simulink model "Progetto"  (R2022b)
settings: Solver=FixedStepDiscrete  StartTime=0.0  StopTime=10.0  FixedStep=0.1  RelTol=1e-3
InitFcn:
  | mbd_s32k_consistency_checks(bdroot(gcs));
libraries: simulink x1, mbd_s32k1xx_ec_toolbox x1
settings Model: Creator=marpe  LastModifiedBy=marpe
settings DataIOCC: ExternalInput=off  InitialState=off  SaveOutput=off  SignalLogging=off  SaveTime=off
settings OptimizationCC: DefaultParameterBehavior=Inlined  EnhancedBackFolding=on  PassReuseOutputArgsAs=Individual arguments  ZeroExternalMemoryAtStartup=off  ZeroInternalMemoryAtStartup=off  OptimizeBlockOrder=speed  DifferentSizesBufferReuse=on  OptimizationCustomize=off  EfficientTunableParamExpr=on
settings DebuggingCC: InheritedTsInSrcMsg=none  SingleTaskRateTransMsg=error  ParameterTunabilityLossMsg=error  UnconnectedInputMsg=error  UnconnectedOutputMsg=error  UnconnectedLineMsg=error  UnknownTsInhSupMsg=error
settings HardwareCC: ProdBitPerPointer=32  ProdBitPerSizeT=32  ProdBitPerPtrDiffT=32  ProdLargestAtomicInteger=Long  ProdLargestAtomicFloat=Double  ProdWordSize=32  ProdHWDeviceType=ARM Compatible->ARM Cortex
settings ModelReferenceCC: ModelReferenceNumInstancesAllowed=Single  PropagateVarSize=During execution
settings SFSimCC: MATLABDynamicMemAlloc=off
settings RTWCC: Description=Model Based Design Toolbox S32K1xx Code Generation Target  SystemTargetFile=mbd_s32k.tlc  MakeCommand=mbd_s32k_make_rtw COPY_MDLREF_INCLUDES=0  TemplateMakefile=mbd_s32k.tmf  GenerateReport=on  LaunchReport=on  GenerateWebview=on
settings CodeAppCC: ForceParamTrailComments=on  IgnoreCustomStorageClasses=off  OperatorAnnotations=on  SimulinkDataObjDesc=on  SFDataObjDesc=on  InsertBlockDesc=on
settings STFCustomTargetCC: TargetLangStandard=C99 (ISO)  MultiwordLength=256  CombineOutputUpdateFcns=on  ERTCustomFileBanners=on  SupportContinuousTime=off  SupportNonInlinedSFcns=off  RemoveResetFunc=on  SupportVariableSizeSignals=on  MATLABClassNameForMDSCustomization=Simulink.SoftwareTarget.ERTCustomization  SystemTargetFile=mbd_s32k.tlc
settings ERTTargetCC: TargetLangStandard=C99 (ISO)  ParMdlRefBuildCompliant=off  CompOptLevelCompliant=off  ConcurrentExecutionCompliant=off  SupportVariableSizeSignals=on  ModelStepFunctionPrototypeControlCompliant=off  CPPClassGenCompliant=off  UseToolchainInfoCompliant=off  InlinedParameterPlacement=NonHierarchical  ERTSrcFileBannerTemplate=mbd_ert_code_template.cgt  ERTHdrFileBannerTemplate=mbd_ert_code_template.cgt  ERTDataSrcFileTemplate=mbd_ert_code_template.cgt  ERTDataHdrFileTemplate=mbd_ert_code_template.cgt  ERTCustomFileTemplate=example_file_process.tlc

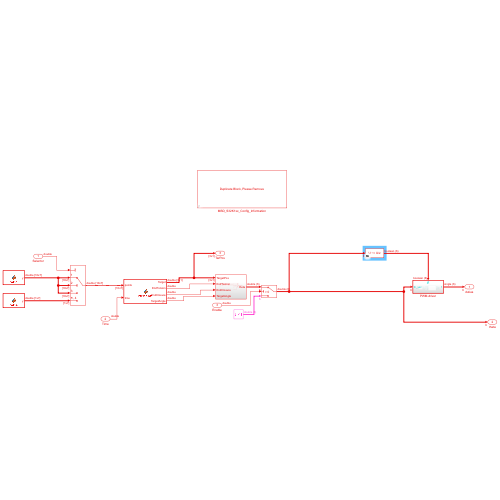
[thumbnail: Simulink's stored preview of the top-level diagram]
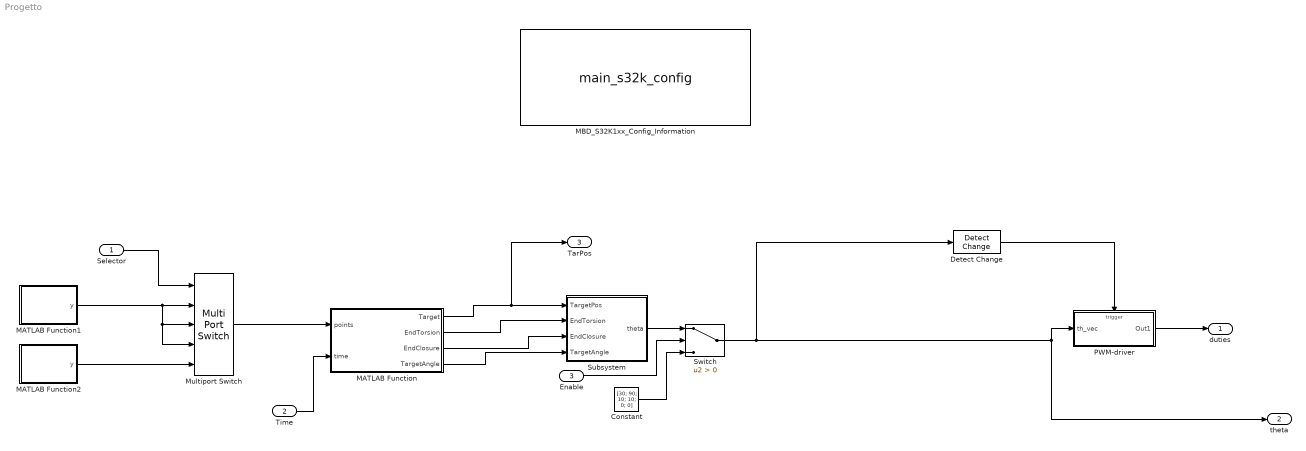
== system Progetto ==
  Selector : Inport  PortDimensions=1
  Time : Inport  Port=2  PortDimensions=1
  Enable : Inport  Port=3
  Constant : Constant  Value=[30; 90; 10; 10; 0; 0]
  Detect Change : simulink/Logic and Bit Operations/Detect Change  vinit=[0; 0; 0; 0; 0; 0]  OutDataTypeStr=boolean
  MATLAB Function : MATLAB Function  TreatAsAtomicUnit=on
  MATLAB Function1 : MATLAB Function  TreatAsAtomicUnit=on
  MATLAB Function2 : MATLAB Function  TreatAsAtomicUnit=on
  MBD_S32K1xx_Config_Information : S-Function  AncestorBlock=mbd_s32k1xx_ec_toolbox/MBD_S32K1xx_Config_Information  LoadFcn=|  InitFcn=|  FunctionName=main_s32k_config  SFunctionDeploymentMode=off  EnableBusSupport=off  mask(MBDTBX_EC_S32K){mbdt_ver=0, disp_str=|, config_params=[], mcu_target_name=S32K144, mcu_target_package=100-LQFP, mcu_target_sram_size=48KB, mcu_system_clock_freq=80, mcu_xtal_freq=External 8, mcu_steptick_timer=LPIT Channel 0, mcu_steptick_prio=15, ds_import_enable=on, target_compiler=GCC, target_memory=FLASH, gcc_target_compile_opts=-mthumb -mfloat-abi=hard -mfpu=fpv4-sp-d16 -O1 -g -gstrict-dwarf, gcc_target_assemble_opts=-mthumb -mfloat-abi=hard -mfpu=fpv4-sp-d16 -g, gcc_target_link_opts=-mthumb -mfloat-abi=hard -mfpu=fpv4-sp-d16, gcc_target_lib_opts=, gcc_target_default_lcf=on, gcc_target_user_lcf=S32K144_48_flash.ld, ghs_target_compile_opts=-cpu=cortexm4f -thumb -fpu=vfpv4_d16 -fsingle -Ogeneral -Wundef -Wimplicit-int -Wshadow -Wtrigraphs --no_commons --gnu_asm -gnu99 -gdwarf-2 -G, ghs_target_assemble_opts=-cpu=cortexm4f -fpu=vfpv4_d16, ghs_target_link_opts=-cpu=cortexm4f -thumb -fpu=vfpv4_d16, ghs_target_lib_opts=, ghs_target_default_lcf=on, ghs_target_user_lcf=S32K144_48_flash.ld, iar_target_compile_opts=--cpu=Cortex-M4F --thumb --fpu=VFPv4_sp -Ol -e --debug --dlib_config normal, iar_target_assemble_opts=--cpu Cortex-M4F --thumb --fpu VFPv4_sp, iar_target_link_opts=--no_exceptions --vfe --inline, iar_target_lib_opts=, iar_target_default_lcf=on, iar_target_user_lcf=S32K144_48_flash.icf, pil_download_enable=on, rbl_download_enable=on, rbl_start_delay=5000, rbl_download_interface=OpenSDA, rbl_restart_request=off, rbl_com_port=COM12, rbl_com_port_custom=COM1, pil_download_rate=115200, pil_download_rate_custom=115200, pil_opensda_drive=Custom, pil_opensda_drive_custom=D, jtag_interface=OpenSDA Embedded Debug, jlink_default_path=on, jlink_user_path=C:\Program Files\SEGGER\JLink\, pil_uart_instance=1, pil_uart_rx=PTC6: [LPUART1_RX | Receive], pil_uart_tx=PTC7: [LPUART1_TX | Transmit], FTM_PWM_PcrCheckEnDis=on, FTM_Input_Edge_Inputs_PcrCheckEnDis=on, FTM_Dual_Edge_Inputs_PcrCheckEnDis=on, FTM_Quadrature_Inputs_PcrCheckEnDis=on, FTM_Hall_Sensor_Inputs_PcrCheckEnDis=on, LPTMR_PcrCheckEnDis=on, PIT_PcrCheckEnDis=on, RTC_PcrCheckEnDis=on, FlexCAN_PcrCheckEnDis=on, LIN_PcrCheckEnDis=on, FlexIO_PcrCheckEnDis=on, LPI2C_PcrCheckEnDis=on, LPSPI_PcrCheckEnDis=on, LPUART_PcrCheckEnDis=on, CMP_PcrCheckEnDis=on, GPIO_OutputPcrCheckEnDis=on, GPIO_InputPcrCheckEnDis=on, SBC_PcrCheckEnDis=on, BMS_PcrCheckEnDis=on, AMMCLIB_PcrCheckEnDis=on, FM_PcrCheckEnDis=on, Profile_PcrCheckEnDis=on, ConfigParams_PcrCheckEnDis=on, ModelRef_PcrCheckEnDis=on, PDB0_PcrCheckEnDis=on, CSEc_PcrCheckEnDis=on, eDMA_PcrCheckEnDis=on, FLASH_PcrCheckEnDis=on, ADC_PcrCheckEnDis=on, WDOG_PcrCheckEnDis=on}
      LoadFcn=|
      | mbd_s32k_set_cur_model(bdroot(gcs));
      | mbd_s32k_block_load(bdroot(gcs));
      InitFcn=|
      | mbd_s32k_set_cur_model(bdroot(gcs)); 
      | mbd_s32k_update_model('init');       
      | mbd_s32k_check('MBDTBX_EC_S32K14');
      mask disp_str=|
      | Target : S32K144-64KB_SRAM
      | Package : 100-pin
      | System clock : 80 MHz
      | XTAL clock : External 8 MHz
      | Compiler : IAR
      | Target Type : FLASH
      | Download Code after build : off
      | Step Tick Interrupt Priority : 15
      mask prompts: mbdt_ver "MBDT Version"; disp_str "display_string"; mcu_target_name "Family"; mcu_target_package "Package"; mcu_target_sram_size "SRAM"; mcu_system_clock_freq "Clock Frequency MHz"; mcu_xtal_freq "XTAL Frequency MHz"; mcu_steptick_timer "Timer"; mcu_steptick_prio "Priority"; ds_import_enable "Generate S32 Design Studio ProjectInfo.xml file"; target_compiler "Compiler"; target_memory "Target Memory Model"; gcc_target_compile_opts "Compile Options"; gcc_target_assemble_opts "Assemble Options"; gcc_target_link_opts "Link Options"; gcc_target_lib_opts "Library Options"; gcc_target_default_lcf "Default Target Memory Definitions"; gcc_target_user_lcf "User Defined Target Memory Definitions"; ghs_target_compile_opts "Compile Options"; ghs_target_assemble_opts "Assemble Options"; ghs_target_link_opts "Link Options"; ghs_target_lib_opts "Library Options"; ghs_target_default_lcf "Default Target Memory Definitions"; ghs_target_user_lcf "User Defined Target Memory Definitions"; iar_target_compile_opts "Compile Options"; iar_target_assemble_opts "Assemble Options"; iar_target_link_opts "Link Options"; iar_target_lib_opts "Library Options"; iar_target_default_lcf "Default Target Memory Definitions"; iar_target_user_lcf "User Defined Target Memory Definitions"; pil_download_enable "Processor-in-the-Loop (PIL) Mode Download"; rbl_download_enable "Download Code after Build"; rbl_start_delay "Delay before start of application (ms)"; rbl_download_interface "Download Interface"; rbl_restart_request "Boot Assist Module (BAM) Restart Request"; rbl_com_port "COM Port"; rbl_com_port_custom "Custom COM Port"; pil_download_rate "Baud Rate"; pil_download_rate_custom "Custom baud rate"; pil_opensda_drive "OpenSDA Drive Name"; pil_opensda_drive_custom "Custom OpenSDA Drive Name"; jtag_interface "Interface"; jlink_default_path "Default JLink installation path"; jlink_user_path "SEGGER JLink installation path"; pil_uart_instance "LPUART"; pil_uart_rx "RX pin"; pil_uart_tx "TX pin"; FTM_PWM_PcrCheckEnDis "FTM PWM Config"; FTM_Input_Edge_Inputs_PcrCheckEnDis "FTM Input Edge Inputs"; FTM_Dual_Edge_Inputs_PcrCheckEnDis "FTM Dual Edge Inputs"; FTM_Quadrature_Inputs_PcrCheckEnDis "FTM Quadrature Inputs"; FTM_Hall_Sensor_Inputs_PcrCheckEnDis "FTM Hall Sensor Inputs"; LPTMR_PcrCheckEnDis "LPTMR"; PIT_PcrCheckEnDis "PIT"; RTC_PcrCheckEnDis "RTC"; FlexCAN_PcrCheckEnDis "FlexCAN"; LIN_PcrCheckEnDis "LIN"; FlexIO_PcrCheckEnDis "FlexIO"; LPI2C_PcrCheckEnDis "LPI2C"; LPSPI_PcrCheckEnDis "LPSPI"; LPUART_PcrCheckEnDis "LPUART"; CMP_PcrCheckEnDis "CMP"; GPIO_OutputPcrCheckEnDis "GPIO Output"; GPIO_InputPcrCheckEnDis "GPIO Input"; SBC_PcrCheckEnDis "SBC"; BMS_PcrCheckEnDis "BMS"; AMMCLIB_PcrCheckEnDis "AMMCLIB"; FM_PcrCheckEnDis "FreeMaster"; Profile_PcrCheckEnDis "Profile"; ConfigParams_PcrCheckEnDis "Config Params"; ModelRef_PcrCheckEnDis "Model Reference"; PDB0_PcrCheckEnDis "PDB"; CSEc_PcrCheckEnDis "CSEc"; eDMA_PcrCheckEnDis "eDMA"; FLASH_PcrCheckEnDis "FLASH"; ADC_PcrCheckEnDis "ADC"; WDOG_PcrCheckEnDis "WDOG"
      mask help: Model-Based Design Toolbox Config block for S32K1xx family of processors.
      mask init:
      | mbd_s32k_config_com_ports_cbk('populate_drop_down');
      | maskStr = mbd_s32k_mb_display_string();
      settings: LibrarySourceBlock=mbd_s32k1xx_ec_toolbox/MBD_S32K1xx_Config_Information  NameChangeFcn=mbd_s32k_model_close;
      settings: CopyFcn=|
      | mbd_s32k_set_cur_model(bdroot(gcs));
      | mbd_s32k_check('MBDTBX_EC_S32K');
      | mbd_s32k_update_model('copy');
      settings: ModelCloseFcn=|
      | mbd_s32k_set_cur_model(bdroot(gcs));
      | mbd_s32k_model_close;
      settings: CloseFcn=|
      | mbd_s32k_set_cur_model(bdroot(gcs));
      | mbd_s32k_check('MBDTBX_EC_S32K');
      | mbd_s32k_update_model('copy');
      mask Help: web(fullfile(mbd_s32k_block_help, 'main_config', 'main_config.html'));
      mask TypeOptions mcu_target_name: S32K116 | S32K118 | S32K142 | S32K144 | S32K146 | S32K148 | S32K142W | S32K144W
      mask Callback mcu_target_name:
      | mbd_s32k_config_target_cbk('mcu_target_name');
      | mbd_s32k_config_target_cbk('mcu_target_compiler');
      | mbd_s32k_config_target_cbk('mcu_target_memory');
      mask TypeOptions mcu_target_package: 48-LQFP | 64-LQFP | 100-LQFP | 100-BGA
      mask Callback mcu_target_package: mbd_s32k_config_target_cbk('mcu_target_package')
      mask TypeOptions mcu_target_sram_size: 48KB | 64KB
      mask Callback mcu_target_sram_size: mbd_s32k_config_target_cbk('mcu_target_sram_size')
      mask TypeOptions mcu_system_clock_freq: 80 | 112
      mask TypeOptions mcu_xtal_freq: External 8 | External 16 | External 24 | External 32 | External 40
      mask TypeOptions mcu_steptick_timer: LPIT Channel 0 | Suppress
      mask TypeOptions mcu_steptick_prio: 15 | 14 | 13 | 12 | 11 | 10 | 9 | 8 | 7 | 6 | 5 | 4 | 3 | 2 | 1 | 0
      mask TypeOptions target_compiler: GCC | IAR | GreenHills Multi
      mask Callback target_compiler: mbd_s32k_config_compiler_cbk('target_compiler')
      mask TypeOptions target_memory: FLASH | SRAM
      mask Callback target_memory: mbd_s32k_config_memory_cbk('target_memory')
      mask Callback gcc_target_default_lcf: mbd_s32k_config_lcf_cbk('gcc_target_default_lcf')
      mask TypeOptions gcc_target_user_lcf: S32K144_48_flash.ld | S32K144_48_flash_bam.ld
      mask Callback ghs_target_default_lcf: mbd_s32k_config_lcf_cbk('ghs_target_default_lcf')
      mask TypeOptions ghs_target_user_lcf: S32K144_48_flash.ld | S32K144_48_flash_bam.ld
      mask Callback iar_target_default_lcf: mbd_s32k_config_lcf_cbk('iar_target_default_lcf')
      mask TypeOptions iar_target_user_lcf: S32K144_48_flash.icf | S32K144_48_flash_bam.icf
      mask Callback pil_download_enable: mbd_s32k_config_pil_cbk('pil_download_enable')
      mask Callback rbl_download_enable: mbd_s32k_config_pil_cbk('rbl_download_enable');
      mask TypeOptions rbl_download_interface: Serial | OpenSDA | JTAG
      mask Callback rbl_download_interface: mbd_s32k_config_pil_cbk('rbl_download_interface')
      mask TypeOptions rbl_com_port: COM12 | Custom
      mask Callback rbl_com_port: mbd_s32k_config_com_ports_cbk('populate_drop_down')
      mask TypeOptions pil_download_rate: 9600 | 14400 | 19200 | 38400 | 56000 | 57600 | 115200 | 128000 | 256000 | 512000 | Custom
      mask Callback pil_download_rate: mbd_s32k_config_pil_cbk('pil_download_rate');
      mask TypeOptions pil_opensda_drive: D: EVB-S32K144 | Custom
      mask Callback pil_opensda_drive:
      | mbd_s32k_config_vol_disks_cbk('populate_drop_down');
      | mbd_s32k_config_vol_disks_cbk('enable_custom');
      mask TypeOptions jtag_interface: OpenSDA Embedded Debug | USB Multilink PEmicro | SEGGER JLink
      mask Callback jtag_interface: mbd_s32k_config_pil_cbk('jtag_interface')
      mask Callback jlink_default_path: mbd_s32k_config_jlink_path
      mask TypeOptions pil_uart_instance: 0 | 1 | 2
      mask Callback pil_uart_instance: mbd_s32k_config_pil_cbk('pil_uart_instance');
      mask TypeOptions pil_uart_rx: PTC6: [LPUART1_RX | Receive] | PTC8: [LPUART1_RX | Receive] | PTD13: [LPUART1_RX | Receive]
      mask TypeOptions pil_uart_tx: PTC7: [LPUART1_TX | Transmit] | PTC9: [LPUART1_TX | Transmit] | PTD14: [LPUART1_TX | Transmit]
      mask DialogControl mcu_config_tab Prompt: MCU
      mask DialogControl Container14 Prompt: Target MCU
      mask DialogControl Container15 Prompt: Clock
      mask DialogControl Container16 Prompt: Step Tick
      mask DialogControl propagate_configuration Prompt: Propagate configuration
      mask DialogControl propagate_configuration Callback: mbd_s32k_config_propagate_cbk(gcb);
      mask DialogControl Container11 Prompt: Build Toolchain
      mask DialogControl Container19 Prompt: General Settings
      mask DialogControl container_GCC Prompt: GCC
      mask DialogControl container_GHS Prompt: GreenHills Multi
      mask DialogControl container_IAR Prompt: IAR
      mask DialogControl Container13 Prompt: Target Connection
      mask DialogControl Container22 Prompt: Mode
      mask DialogControl Container22_copy Prompt: Download settings
      mask DialogControl Container23 Prompt: Serial
      mask DialogControl rbl_com_button Prompt: Refresh
      mask DialogControl rbl_com_button Callback: mbd_s32k_config_com_ports_cbk('populate_drop_down')
      mask DialogControl Container26 Prompt: OpenSDA
      mask DialogControl pil_opensda_refresh Prompt: Refresh
      mask DialogControl pil_opensda_refresh Callback: mbd_s32k_config_vol_disks_cbk('populate_drop_down')
      mask DialogControl Container39 Prompt: JTAG
      mask DialogControl PIL_Settings_Container Prompt: PIL Settings
      mask DialogControl Container12 Prompt: Diagnostics
      mask DialogControl Container17 Prompt: Consistency checks
      mask DialogControl Container28 Prompt: Timers
      mask DialogControl Container30 Prompt: Communication
      mask DialogControl Container34 Prompt: Analog and Digital
      mask DialogControl Container18 Prompt: Utilities
      mask DialogControl Container33 Prompt: Core and System
      mask Display: disp('Duplicate Block, Please Remove')
  Multiport Switch : MultiPortSwitch  Inputs=4  AllowDiffInputSizes=on  SaturateOnIntegerOverflow=off  InputSameDT=off
  PWM-driver : Subsystem  TreatAsAtomicUnit=on
  Subsystem : Subsystem
  Switch : Switch  Criteria=u2 > Threshold  SaturateOnIntegerOverflow=off  InputSameDT=off
  duties : Outport
  theta : Outport  Port=2
  TarPos : Outport  Port=3
  wires:
  PWM-driver/1(Out1) -> duties/1
  MATLAB Function/1(Target) -> TarPos/1, Subsystem/1(TargetPos)
  MATLAB Function/2(EndTorsion) -> Subsystem/2(EndTorsion)
  MATLAB Function/3(EndClosure) -> Subsystem/3(EndClosure)
  Multiport Switch/1 -> MATLAB Function/1(points)
  Selector/1 -> Multiport Switch/1
  Time/1 -> MATLAB Function/2(time)
  MATLAB Function2/1(y) -> Multiport Switch/5
  MATLAB Function1/1(y) -> Multiport Switch/4, Multiport Switch/3, Multiport Switch/2
  MATLAB Function/4(TargetAngle) -> Subsystem/4(TargetAngle)
  Switch/1 -> Detect Change/1, theta/1, PWM-driver/1(th_vec)
  Subsystem/1(theta) -> Switch/1
  Constant/1 -> Switch/3
  Enable/1 -> Switch/2
  Detect Change/1 -> PWM-driver/Trigger

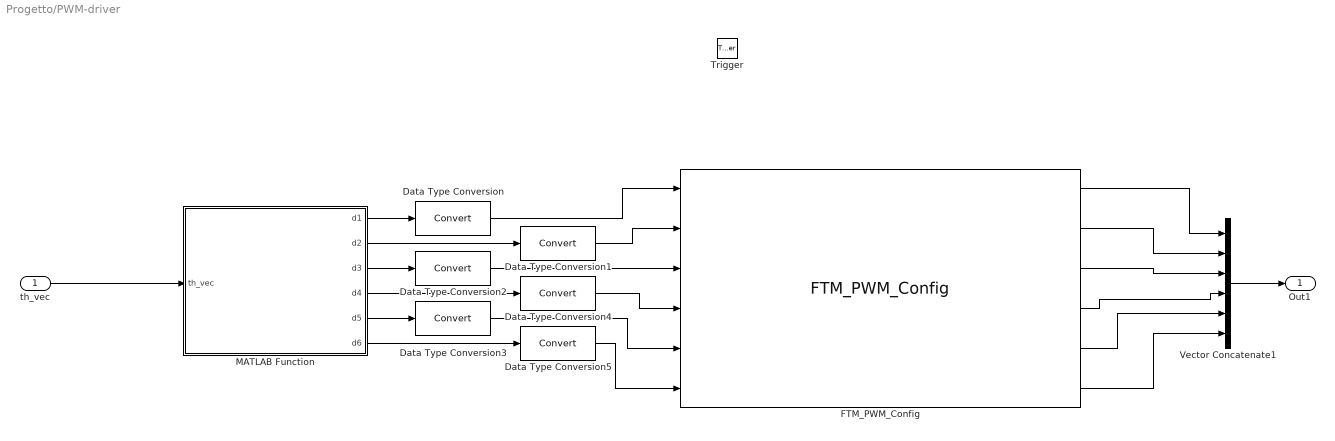
== system Progetto/PWM-driver ==
  th_vec : Inport
  Trigger : TriggerPort  VariantControl=(inherit)  PortDimensions=1
  Data Type Conversion{,1..5} (6 alike) : DataTypeConversion  SaturateOnIntegerOverflow=off  RndMeth=Floor
  FTM_PWM_Config : mbd_s32k1xx_ec_toolbox/Motor Control Blocks/FTM Blocks/FTM_PWM_Config  ftmModule=0  ftmMode=Edge-Aligned PWM  ftmSourceClock=80 MHz  swcontrol_enable=off  chan0En=on  chan0Type=Independent  chan2En=on  chan2Type=Independent  chan4En=on  chan4Type=Independent  chan6En=off  chan6Type=Independent  ftmPwmUnits=Hz  outFrequency=50  ftmPeriod=25000  ftmPrescaler=Divide by 64  deadtimeUnits=Nanoseconds  deadtimeNs=0  deadtimeTicks=0  deadtimePrescaler=Divide by 1  dutyCycleCh0=0.25  dutyCycleCh1=0.25  dutyCycleCh2=0.25  dutyCycleCh3=0.25  dutyCycleCh4=0.25  dutyCycleCh5=0.25  dutyCycleCh6=0.25  dutyCycleCh7=0.25  dutyCycleSim=on  startAfterInit=on  showAdvOpt=on  pinFtmCh0=PTB12: [FTM0_CH0 | FTM Channel]  pinFtmCh1=PTB13: [FTM0_CH1 | FTM Channel]  pinPolCh0=Active High  pinPolCh1=Active High  outputComplem0=Main duplicated  outputLevel0=Low  outputLevel1=Low  pinFtmCh2=PTC2: [FTM0_CH2 | FTM Channel]  pinFtmCh3=PTC3: [FTM0_CH3 | FTM Channel]  pinPolCh2=Active High  pinPolCh3=Active High  outputComplem2=Main duplicated  outputLevel2=Low  outputLevel3=Low  pinFtmCh4=PTB4: [FTM0_CH4 | FTM Channel]  pinFtmCh5=PTB5: [FTM0_CH5 | FTM Channel]  pinPolCh4=Active High  pinPolCh5=Active High  outputComplem4=Main duplicated  outputLevel4=Low  outputLevel5=Low  pinFtmCh6=PTA17: [FTM0_CH6 | FTM Channel]  pinFtmCh7=None  pinPolCh6=Active Low  pinPolCh7=Active Low  outputComplem6=Main duplicated  outputLevel6=Low  outputLevel7=Low  initTrigger=off  chTrigger0=off  chTrigger1=off  chTrigger2=off  chTrigger3=off  chTrigger4=off  chTrigger5=off  chTrigger6=off  chTrigger7=off  mcuTargetUpdate=on  pwmSyncTrg=Software trigger  pwmSyncHwRouting=TRGMUX_FTM7  pwmSyncTrg0=off  pwmSyncTrg1=off  pwmSyncTrg2=off  pwmSyncAutoClear=on  pwmSyncMinLoad=off  pwmSyncMaxLoad=on  pwmSyncInvert=System Clock  pwmSyncOutControl=System Clock  pwmSyncOutMask=System Clock  pwmSyncCounterInitial=System Clock  pwmSyncPoints=Wait Loading Points  reloadEnable=off  reloadPriority=15  reloadHalfCycle=off  reloadHCR=0  reloadFrequency=0  chnMatch0=off  chnMatch1=off  chnMatch2=off  chnMatch3=off  chnMatch4=off  chnMatch5=off  chnMatch6=off  chnMatch7=off  pwmFaultProtection=off  pwmFaultInterrupt=off  pwmFaultClearing=Fault control disabled  pwmFaultPinState=Safe Value  pwmFaultFilterValue=0  pwmFaultPriority=15  fault_disen_0=off  fault_filter_0=off  fault_polarity_0=Active High  fault_disen_1=off  fault_filter_1=off  fault_polarity_1=Active high  fault_disen_2=off  fault_filter_2=off  fault_polarity_2=Active high  fault_disen_3=off  fault_filter_3=off  fault_polarity_3=Active high  fault_pin_0=None  fault_pin_1=None  fault_pin_2=None  fault_pin_3=None
  MATLAB Function : MATLAB Function  TreatAsAtomicUnit=on
  Vector Concatenate1 : Concatenate  NumInputs=6
  Out1 : Outport
  wires:
  FTM_PWM_Config/3 -> Vector Concatenate1/3
  Data Type Conversion1/1 -> FTM_PWM_Config/2
  MATLAB Function/5(d5) -> Data Type Conversion3/1
  FTM_PWM_Config/4 -> Vector Concatenate1/4
  FTM_PWM_Config/2 -> Vector Concatenate1/2
  MATLAB Function/1(d1) -> Data Type Conversion/1
  Vector Concatenate1/1 -> Out1/1
  th_vec/1 -> MATLAB Function/1(th_vec)
  Data Type Conversion5/1 -> FTM_PWM_Config/6
  MATLAB Function/4(d4) -> Data Type Conversion4/1
  Data Type Conversion/1 -> FTM_PWM_Config/1
  FTM_PWM_Config/1 -> Vector Concatenate1/1
  FTM_PWM_Config/5 -> Vector Concatenate1/5
  FTM_PWM_Config/6 -> Vector Concatenate1/6
  Data Type Conversion3/1 -> FTM_PWM_Config/5
  Data Type Conversion4/1 -> FTM_PWM_Config/4
  MATLAB Function/6(d6) -> Data Type Conversion5/1
  Data Type Conversion2/1 -> FTM_PWM_Config/3
  MATLAB Function/3(d3) -> Data Type Conversion2/1
  MATLAB Function/2(d2) -> Data Type Conversion1/1

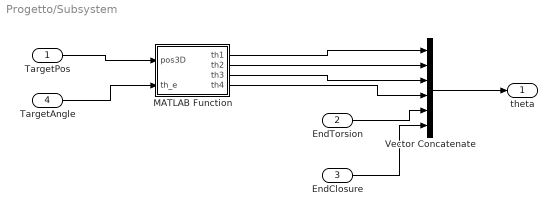
== system Progetto/Subsystem ==
  TargetPos : Inport
  EndTorsion : Inport  Port=2  PortDimensions=1
  EndClosure : Inport  Port=3  PortDimensions=1
  TargetAngle : Inport  Port=4  PortDimensions=1
  MATLAB Function : MATLAB Function  TreatAsAtomicUnit=on
  Vector Concatenate : Concatenate  NumInputs=6
  theta : Outport
  wires:
  EndTorsion/1 -> Vector Concatenate/5
  EndClosure/1 -> Vector Concatenate/6
  Vector Concatenate/1 -> theta/1
  TargetAngle/1 -> MATLAB Function/2(th_e)
  TargetPos/1 -> MATLAB Function/1(pos3D)
  MATLAB Function/1(th1) -> Vector Concatenate/1
  MATLAB Function/2(th2) -> Vector Concatenate/2
  MATLAB Function/3(th3) -> Vector Concatenate/3
  MATLAB Function/4(th4) -> Vector Concatenate/4

== matlab function Progetto/PWM-driver/MATLAB Function ==
  data: th_vec input; d1 output; d2 output; d3 output; d4 output; d5 output; d6 output
function [d1, d2, d3, d4, d5, d6] = angle_to_duty_cycle(th_vec)
    % Angoli in gradi
    lower_limit = [0 15 0 0 0 10];
    upper_limit = [180 165 180 180 180 73];

    % Controllo dei limiti
    th_vec = th_vec.*(th_vec>=lower_limit) + lower_limit.*(th_vec<lower_limit);
    th_vec = th_vec.*(th_vec<=upper_limit) + upper_limit.*(th_vec>upper_limit);

    % Classica interpolazione lineare A(1-alpha)+b(alpha)
    d = (0.5.*(1.-th_vec/180)+2.5.*(th_vec/180))/20;
    % 3 e 1 sono invertiti per qualche motivo
    d1 = d(3);
    d2 = d(2);
    d3 = d(1);
    d4 = d(4);
    d5 = d(5);
    d6 = d(6);

== matlab function Progetto/MATLAB Function ==
  data: points input; Target output; time input; EndTorsion output; EndClosure output; TargetAngle output
function [Target, EndTorsion, EndClosure, TargetAngle] = interpolate(points, time)

    % Ogni punto è una riga, con il tempo alla fine (matrice nx9)
    time_column = size(points, 2);
    n_rows = size(points, 1);
    if (time_column < 7)
        exp_points1 = [points zeros(n_rows, 7-time_column)];
    else
        exp_points1 = points;
    end
    if (n_rows == 1)
        exp_points2 = [exp_points1; (exp_points1+[0 0 0 0 0 0 1])];
    else
        exp_points2 = exp_points1;
    end
    time_instants = exp_points2(:, 7);
    points_at_time = exp_points2(:, 1:6);
    if (time <= time_instants(1, 1))
        point_q = points_at_time(1, :);
    elseif (time >= time_instants(length(time_instants)))
        point_q = points_at_time(length(time_instants), :);
    else
        point_q = interp1(time_instants, points_at_time, time);
    end
    Target = reshape(point_q(1:3), [3, 1]);
    TargetAngle = point_q(4);
    EndTorsion = point_q(5);
    EndClosure = point_q(6);

== matlab function Progetto/Subsystem/MATLAB Function ==
  data: pos3D input; th1 output; th_e input; th2 output; th3 output; th4 output
function [th1, th2, th3, th4] = ik(pos3D, th_e)

% Converti da deg a rad

    th_e = th_e * pi/180;

    L1 = 7;
    L2_3 = 13;
    L4 = 19;

% Sposto tutto su un piano: calcolo th1

    th1 = atan2(pos3D(2), pos3D(1));

% Ruoto pos3D per ottenere le cordinate nel piano

    pos2D = [sqrt(pos3D(1)^2+pos3D(2)^2); pos3D(3)];

% Ottieni coordinate del penultimo giunto dall'orientazione dell'ultimo

    q1 = pos2D(1) - L4*sin(th_e);
    q2 = pos2D(2) - L4*cos(th_e) - L1;

% Ora è uno Scara simmetrico

    cos_angle = 0.5*sqrt(q1^2+q2^2)/L2_3;
    if abs(cos_angle) > 1
        th2 = pi/2 - atan2(q2, q1);
        th3 = 0;
    else
        th2 = pi/2 - atan2(q2, q1) - acos(cos_angle);
        th3 = pi/2 - th2 - atan2(q2-L2_3*cos(th2), q1-L2_3*sin(th2));
    end

% Calcola ultimo angolo

    th4 = th_e - th2 - th3;

    th_vec = [th1, th2, th3, th4];
    th_vec = th_vec * 180/pi;

% Converti agli angoli dei motori
    th_vec = [30, 90, 100, 100] + [th_vec(1), -th_vec(2:4)];

    th_vec = rem(th_vec+360, 360);
    th_vec = th_vec.*(th_vec<=180)+(th_vec-360).*(th_vec>180);
    th1 = th_vec(1);
    th2 = th_vec(2);
    th3 = th_vec(3);
    th4 = th_vec(4);

end

== matlab function Progetto/MATLAB Function1 ==
  data: y output
function y = path1()

    y = [
         9.6    0 10   180  0  0    0;
          18    0  2   180 90  0  500;
          18    0  5   180 90 73 1000;
         9.6    0 10   180 90 73 1500;
           0  9.3 11   180 90 73 2000;
           0   12  9   180 90 73 2500;
           0   18  2   180 90  0 3000;
           0   18  5   180 90  0 3500;
           0   12  9   180 90  0 4000;
         9.6    0 10   180  0  0 4500;
        ];

== matlab function Progetto/MATLAB Function2 ==
  data: y output
function y = path4()

    y = [
         9.6    0 10   180  0  0    0;
        ];
